simulink model "matlab_function_array_test"  (Simulink 8.7)
settings: Solver=FixedStepAuto  StartTime=0.0  StopTime=10.0  RelTol=1e-3
libraries: simulink x4
settings Model: Creator=arnaud  LastModifiedBy=hamza
settings DataIOCC: SaveFormat=Structure
settings DebuggingCC: UnderspecifiedInitializationDetection=Simplified  MergeDetectMultiDrivingBlocksExec=error  SolverPrmCheckMsg=warning
settings ConfigComp: CovSFcnEnable=off

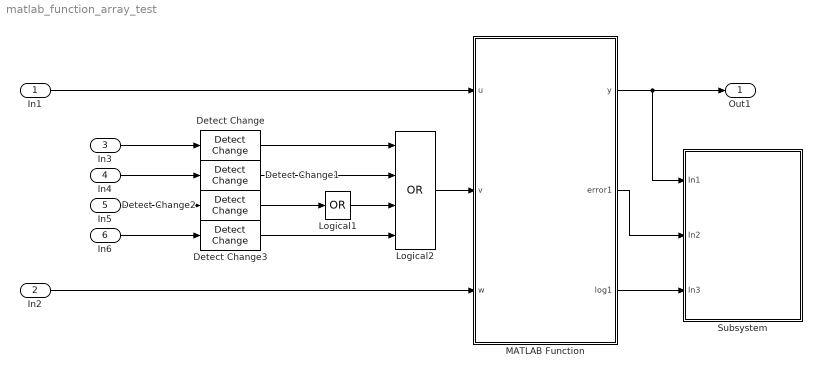
== system matlab_function_array_test ==
  In1 : Inport  OutDataTypeStr=double  PortDimensions=1  BusOutputAsStruct=on
  In2 : Inport  Port=2  OutDataTypeStr=double  PortDimensions=[2 3]
  In3 : Inport  Port=3  OutDataTypeStr=double  PortDimensions=1  BusOutputAsStruct=on
  In4 : Inport  Port=4  OutDataTypeStr=double  PortDimensions=1  BusOutputAsStruct=on
  In5 : Inport  Port=5  OutDataTypeStr=double  PortDimensions=1  BusOutputAsStruct=on
  In6 : Inport  Port=6  OutDataTypeStr=double  PortDimensions=1  BusOutputAsStruct=on
  Detect Change{,1..3} (4 alike) : simulink/Logic and Bit Operations/Detect Change  vinit=0  InputProcessing=Inherited  OutDataTypeStr=boolean
  Logical1 : Logic  Operator=OR  Inputs=1  AllPortsSameDT=off  OutDataTypeStr=boolean
  Logical2 : Logic  Operator=OR  Inputs=4  AllPortsSameDT=off  OutDataTypeStr=boolean
  MATLAB Function : MATLAB Function  TreatAsAtomicUnit=on
  Subsystem : Subsystem  TreatAsAtomicUnit=on
  Out1 : Outport
  wires:
  In1/1 -> MATLAB Function/1(u)
  Logical2/1 -> MATLAB Function/2(v)
  Logical1/1 -> Logical2/3
  Detect Change/1 -> Logical2/1
  Detect Change1/1 -> Logical2/2
  Detect Change2/1 -> Logical1/1
  Detect Change3/1 -> Logical2/4
  In4/1 -> Detect Change1/1
  In3/1 -> Detect Change/1
  In5/1 -> Detect Change2/1
  In6/1 -> Detect Change3/1
  In2/1 -> MATLAB Function/3(w)
  MATLAB Function/1(y) -> Subsystem/1(In1), Out1/1
  MATLAB Function/2(error1) -> Subsystem/2(In2)
  MATLAB Function/3(log1) -> Subsystem/3(In3)

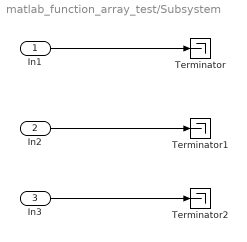
== system matlab_function_array_test/Subsystem ==
  In1 : Inport
  In2 : Inport  Port=2
  In3 : Inport  Port=3
  Terminator : Terminator
  Terminator1 : Terminator
  Terminator2 : Terminator
  wires:
  In1/1 -> Terminator/1
  In2/1 -> Terminator1/1
  In3/1 -> Terminator2/1

== matlab function MATLAB Function ==
  data: u input double; y output double; v input double; w input double; error1 output double; log1 output double
function [y, error1, log1] = do_stuff(u, v, w)
%#codegen

y = u;
error1 = v;
log1 = w;
